simulink model "drone_6dof"  (R2021a)
settings: Solver=VariableStepAuto  StartTime=0.0  StopTime=40  RelTol=1e-3
values from neighbouring files (symbols this model uses):
  controller = designController6DoF(requirements, dynamics)    [mainNelderMead_NOTUSED.m]    (also in mainPSO.m = controllerPre)
  dynamics = getDroneDynamics6DoF()    [mainNelderMead_NOTUSED.m]    (also in mainPSO.m; showResults.m)
undefined symbols (not defined in the file or in its folder): phi0, psi0, theta0, x0, y0, z0
libraries: shared6dof x1
settings Model: SimulationMode=accelerator  Creator=rudog  LastModifiedBy=luizgiacomossi
settings SolverCC: AlgebraicLoopSolver=TrustRegion
settings DebuggingCC: SFMachineParentedDataDiag=warning

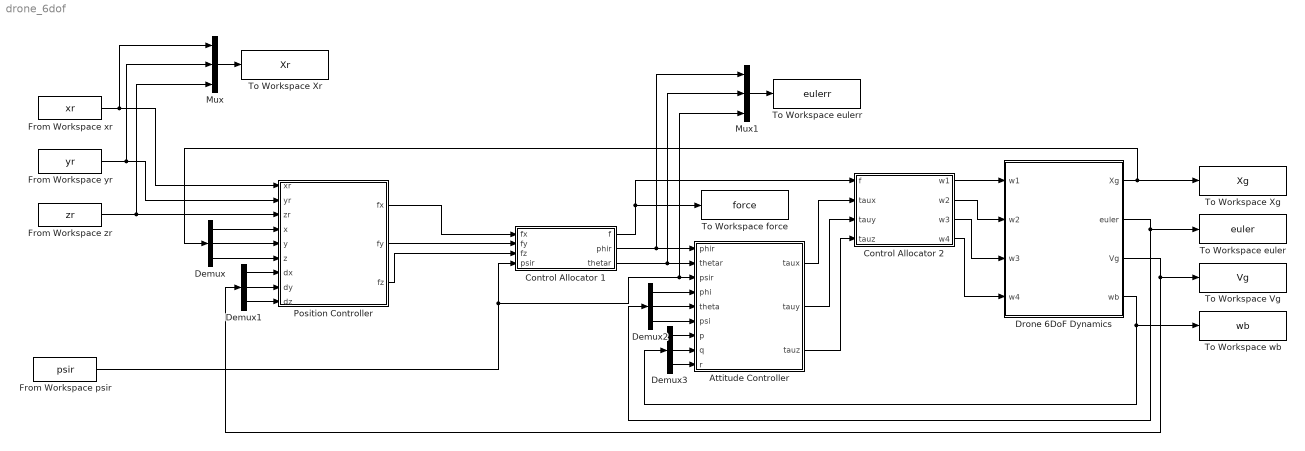
== system drone_6dof ==
  Attitude Controller : Subsystem
  Control Allocator 1 : Subsystem
  Control Allocator 2 : Subsystem
  Demux{,1..3} (4 alike) : Demux  Outputs=3
  Drone 6DoF Dynamics : Subsystem
  From Workspace psir : FromWorkspace  VariableName=psir
  From Workspace xr : FromWorkspace  VariableName=xr
  From Workspace yr : FromWorkspace  VariableName=yr
  From Workspace zr : FromWorkspace  VariableName=zr
  Mux : Mux  Inputs=3
  Mux1 : Mux  Inputs=3
  Position Controller : Subsystem
  To Workspace Vg : ToWorkspace  VariableName=Vg  SaveFormat=Structure With Time  SampleTime=-1
  To Workspace Xg : ToWorkspace  VariableName=Xg  SaveFormat=Structure With Time  SampleTime=-1
  To Workspace Xr : ToWorkspace  VariableName=Xr  SaveFormat=Structure With Time  SampleTime=-1
  To Workspace euler : ToWorkspace  VariableName=euler  SaveFormat=Structure With Time  SampleTime=-1
  To Workspace eulerr : ToWorkspace  VariableName=eulerr  SaveFormat=Structure With Time  SampleTime=-1
  To Workspace force : ToWorkspace  VariableName=force  SaveFormat=Structure With Time  SampleTime=-1
  To Workspace wb : ToWorkspace  VariableName=wb  SaveFormat=Structure With Time  SampleTime=-1
  wires:
  Demux/1 -> Position Controller/4(x)
  Demux/2 -> Position Controller/5(y)
  Demux/3 -> Position Controller/6(z)
  Demux1/1 -> Position Controller/7(dx)
  Demux1/2 -> Position Controller/8(dy)
  Demux1/3 -> Position Controller/9(dz)
  Demux2/1 -> Attitude Controller/4(phi)
  Demux2/2 -> Attitude Controller/5(theta)
  Demux2/3 -> Attitude Controller/6(psi)
  Demux3/1 -> Attitude Controller/7(p)
  Demux3/2 -> Attitude Controller/8(q)
  Demux3/3 -> Attitude Controller/9(r)
  From Workspace zr/1 -> Mux/3, Position Controller/3(zr)
  From Workspace yr/1 -> Mux/2, Position Controller/2(yr)
  From Workspace xr/1 -> Mux/1, Position Controller/1(xr)
  Control Allocator 2/1(w1) -> Drone 6DoF Dynamics/1(w1)
  Control Allocator 2/2(w2) -> Drone 6DoF Dynamics/2(w2)
  Control Allocator 2/3(w3) -> Drone 6DoF Dynamics/3(w3)
  Control Allocator 2/4(w4) -> Drone 6DoF Dynamics/4(w4)
  Control Allocator 1/1(f) -> To Workspace force/1, Control Allocator 2/1(f)
  Attitude Controller/1(taux) -> Control Allocator 2/2(taux)
  Attitude Controller/2(tauy) -> Control Allocator 2/3(tauy)
  Attitude Controller/3(tauz) -> Control Allocator 2/4(tauz)
  Drone 6DoF Dynamics/3(Vg) -> Demux1/1, To Workspace Vg/1
  Drone 6DoF Dynamics/4(wb) -> Demux3/1, To Workspace wb/1
  Mux/1 -> To Workspace Xr/1
  Control Allocator 1/2(phir) -> Mux1/1, Attitude Controller/1(phir)
  Control Allocator 1/3(thetar) -> Mux1/2, Attitude Controller/2(thetar)
  From Workspace psir/1 -> Control Allocator 1/4(psir), Mux1/3, Attitude Controller/3(psir)
  Mux1/1 -> To Workspace eulerr/1
  Position Controller/2(fy) -> Control Allocator 1/2(fy)
  Position Controller/1(fx) -> Control Allocator 1/1(fx)
  Position Controller/3(fz) -> Control Allocator 1/3(fz)
  Drone 6DoF Dynamics/2(euler) -> Demux2/1, To Workspace euler/1
  Drone 6DoF Dynamics/1(Xg) -> To Workspace Xg/1, Demux/1

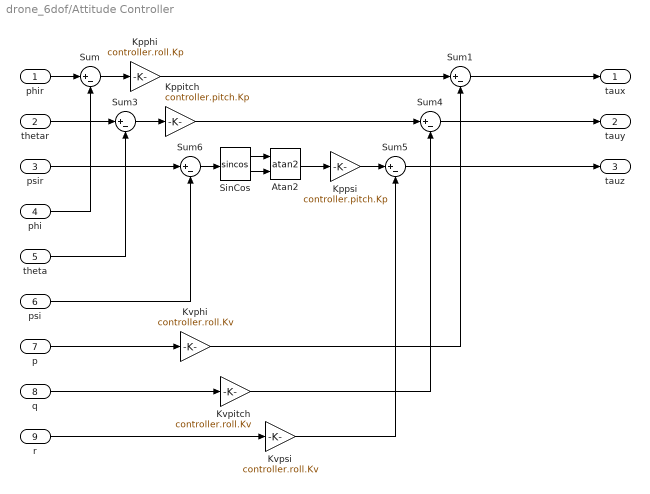
== system drone_6dof/Attitude Controller ==
  phir : Inport
  thetar : Inport  Port=2
  psir : Inport  Port=3
  phi : Inport  Port=4
  theta : Inport  Port=5
  psi : Inport  Port=6
  p : Inport  Port=7
  q : Inport  Port=8
  r : Inport  Port=9
  Atan2 : Trigonometry  Operator=atan2
  Kpphi : Gain  Gain=controller.roll.Kp
  Kppitch : Gain  Gain=controller.pitch.Kp
  Kppsi : Gain  Gain=controller.pitch.Kp
  Kvphi : Gain  Gain=controller.roll.Kv
  Kvpitch : Gain  Gain=controller.roll.Kv
  Kvpsi : Gain  Gain=controller.roll.Kv
  SinCos : Trigonometry  Operator=sincos
  Sum{,1,3..6} (6 alike) : Sum  Inputs=|+-
  taux : Outport
  tauy : Outport  Port=2
  tauz : Outport  Port=3
  wires:
  Kvphi/1 -> Sum1/2
  p/1 -> Kvphi/1
  Kppsi/1 -> Sum5/1
  Sum3/1 -> Kppitch/1
  theta/1 -> Sum3/2
  phir/1 -> Sum/1
  SinCos/1 -> Atan2/1
  Sum1/1 -> taux/1
  Kppitch/1 -> Sum4/1
  Kvpitch/1 -> Sum4/2
  Sum4/1 -> tauy/1
  Kpphi/1 -> Sum1/1
  q/1 -> Kvpitch/1
  r/1 -> Kvpsi/1
  psi/1 -> Sum6/2
  psir/1 -> Sum6/1
  Sum6/1 -> SinCos/1
  SinCos/2 -> Atan2/2
  Sum5/1 -> tauz/1
  Kvpsi/1 -> Sum5/2
  thetar/1 -> Sum3/1
  Atan2/1 -> Kppsi/1
  phi/1 -> Sum/2
  Sum/1 -> Kpphi/1

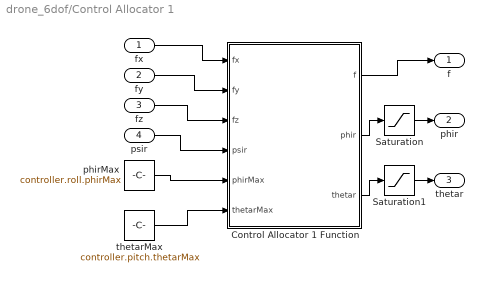
== system drone_6dof/Control Allocator 1 ==
  fx : Inport
  fy : Inport  Port=2
  fz : Inport  Port=3
  psir : Inport  Port=4
  Control Allocator 1 Function : MATLAB Function  TreatAsAtomicUnit=on
  Saturation : Saturate  UpperLimit=30 * pi/180  LowerLimit=- 30 * pi/180
  Saturation1 : Saturate  UpperLimit=30 * pi/180  LowerLimit=- 30 * pi/180
  phirMax : Constant  Value=controller.roll.phirMax
  thetarMax : Constant  Value=controller.pitch.thetarMax
  f : Outport
  phir : Outport  Port=2
  thetar : Outport  Port=3
  wires:
  fx/1 -> Control Allocator 1 Function/1(fx)
  fy/1 -> Control Allocator 1 Function/2(fy)
  fz/1 -> Control Allocator 1 Function/3(fz)
  psir/1 -> Control Allocator 1 Function/4(psir)
  Control Allocator 1 Function/1(f) -> f/1
  Control Allocator 1 Function/2(phir) -> Saturation/1
  Control Allocator 1 Function/3(thetar) -> Saturation1/1
  phirMax/1 -> Control Allocator 1 Function/5(phirMax)
  thetarMax/1 -> Control Allocator 1 Function/6(thetarMax)
  Saturation/1 -> phir/1
  Saturation1/1 -> thetar/1

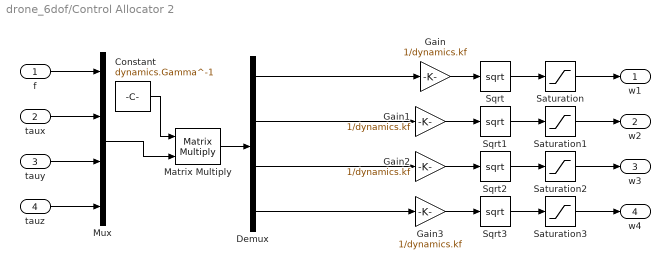
== system drone_6dof/Control Allocator 2 ==
  f : Inport
  taux : Inport  Port=2
  tauy : Inport  Port=3
  tauz : Inport  Port=4
  Constant : Constant  Value=dynamics.Gamma^-1
  Demux : Demux
  Gain{,1..3} (4 alike) : Gain  Gain=1/dynamics.kf
  Matrix Multiply : Product  Multiplication=Matrix(*)
  Mux : Mux
  Saturation{,1..3} (4 alike) : Saturate  UpperLimit=dynamics.wMax  LowerLimit=dynamics.wMin
  Sqrt{,1..3} (4 alike) : Sqrt  SaturateOnIntegerOverflow=on
  w1 : Outport
  w2 : Outport  Port=2
  w3 : Outport  Port=3
  w4 : Outport  Port=4
  wires:
  Gain/1 -> Sqrt/1
  Gain1/1 -> Sqrt1/1
  Gain2/1 -> Sqrt2/1
  Gain3/1 -> Sqrt3/1
  Sqrt3/1 -> Saturation3/1
  Sqrt2/1 -> Saturation2/1
  Sqrt1/1 -> Saturation1/1
  Sqrt/1 -> Saturation/1
  Saturation/1 -> w1/1
  Saturation1/1 -> w2/1
  Saturation2/1 -> w3/1
  Saturation3/1 -> w4/1
  Demux/2 -> Gain1/1
  Demux/4 -> Gain3/1
  Demux/3 -> Gain2/1
  f/1 -> Mux/1
  taux/1 -> Mux/2
  tauy/1 -> Mux/3
  tauz/1 -> Mux/4
  Constant/1 -> Matrix Multiply/1
  Mux/1 -> Matrix Multiply/2
  Matrix Multiply/1 -> Demux/1
  Demux/1 -> Gain/1

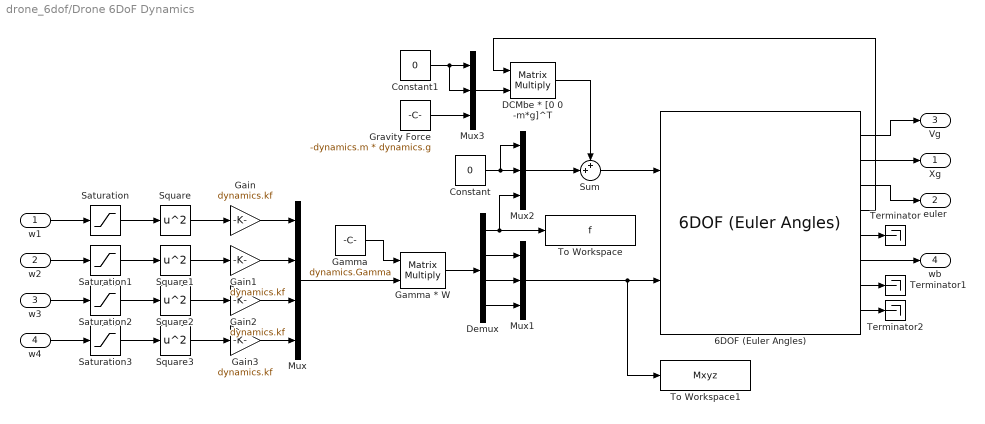
== system drone_6dof/Drone 6DoF Dynamics ==
  w1 : Inport
  w2 : Inport  Port=2
  w3 : Inport  Port=3
  w4 : Inport  Port=4
  6DOF (Euler Angles) : shared6dof/6DOF (Euler Angles)  units=Metric (MKS)  mtype=Fixed  rep=Euler Angles  xme_0=[x0, y0, z0]  Vm_0=[0 0 0]  eul_0=[phi0, theta0, psi0]  pm_0=[0 0 0]  mass_0=dynamics.m  mass_e=0.5  mass_f=2.0  inertia=dynamics.J  inertia_e=eye(3)  inertia_f=2*eye(3)  k_quat=1.0  vre_flag=on  abi_flag=off  aMode=0  xme_statename=''  Vm_statename=''  eul_statename=''  quat_statename=''  pm_statename=''  mass_statename=''
      settings: SourceProductBaseCode=AE,PW,DR,MT,UV,VE
  Constant : Constant  Value=0
  Constant1 : Constant  Value=0
  DCMbe * [0 0 -m*g]^T : Product  Multiplication=Matrix(*)
  Demux : Demux
  Gain{,1..3} (4 alike) : Gain  Gain=dynamics.kf
  Gamma : Constant  Value=dynamics.Gamma
  Gamma * W : Product  Multiplication=Matrix(*)
  Gravity Force : Constant  Value=-dynamics.m * dynamics.g
  Mux : Mux
  Mux1 : Mux  Inputs=3
  Mux2 : Mux  Inputs=3
  Mux3 : Mux  Inputs=3
  Saturation{,1..3} (4 alike) : Saturate  UpperLimit=dynamics.wMax  LowerLimit=dynamics.wMin
  Square{,1..3} (4 alike) : Math  Operator=square  SaturateOnIntegerOverflow=on
  Sum : Sum  Inputs=++|
  Terminator : Terminator
  Terminator1 : Terminator
  Terminator2 : Terminator
  To Workspace : ToWorkspace  VariableName=f  SaveFormat=Structure With Time  SampleTime=-1
  To Workspace1 : ToWorkspace  VariableName=Mxyz  SaveFormat=Structure With Time  SampleTime=-1
  Xg : Outport
  euler : Outport  Port=2
  Vg : Outport  Port=3
  wb : Outport  Port=4
  wires:
  6DOF (Euler Angles)/2 -> Xg/1
  6DOF (Euler Angles)/1 -> Vg/1
  6DOF (Euler Angles)/3 -> euler/1
  w1/1 -> Saturation/1
  w2/1 -> Saturation1/1
  w3/1 -> Saturation2/1
  w4/1 -> Saturation3/1
  Gamma * W/1 -> Demux/1
  Demux/2 -> Mux1/1
  Demux/3 -> Mux1/2
  Demux/4 -> Mux1/3
  Mux1/1 -> To Workspace1/1, 6DOF (Euler Angles)/2
  Mux/1 -> Gamma * W/2
  Gamma/1 -> Gamma * W/1
  Constant/1 -> Mux2/1, Mux2/2
  Demux/1 -> Mux2/3, To Workspace/1
  Mux2/1 -> Sum/2
  Sum/1 -> 6DOF (Euler Angles)/1
  6DOF (Euler Angles)/6 -> wb/1
  6DOF (Euler Angles)/5 -> Terminator/1
  6DOF (Euler Angles)/7 -> Terminator1/1
  6DOF (Euler Angles)/8 -> Terminator2/1
  Gravity Force/1 -> Mux3/3
  Mux3/1 -> DCMbe * [0 0 -m*g]^T/2
  6DOF (Euler Angles)/4 -> DCMbe * [0 0 -m*g]^T/1
  Constant1/1 -> Mux3/2, Mux3/1
  DCMbe * [0 0 -m*g]^T/1 -> Sum/1
  Saturation/1 -> Square/1
  Square/1 -> Gain/1
  Gain/1 -> Mux/1
  Gain1/1 -> Mux/2
  Saturation1/1 -> Square1/1
  Saturation2/1 -> Square2/1
  Saturation3/1 -> Square3/1
  Square1/1 -> Gain1/1
  Square2/1 -> Gain2/1
  Square3/1 -> Gain3/1
  Gain2/1 -> Mux/3
  Gain3/1 -> Mux/4

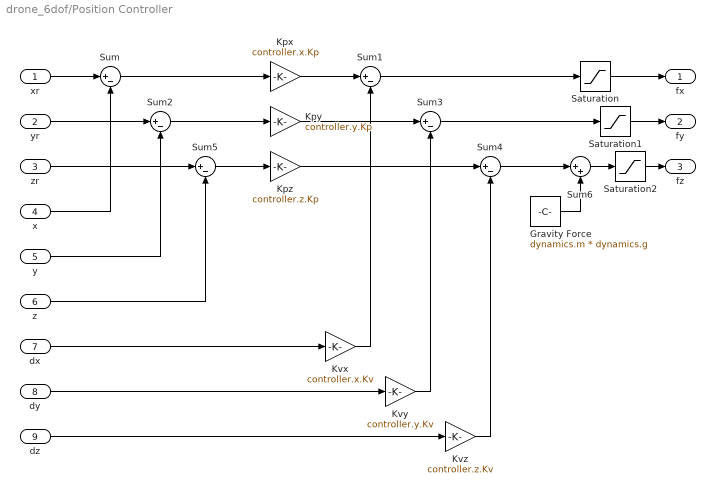
== system drone_6dof/Position Controller ==
  xr : Inport
  yr : Inport  Port=2
  zr : Inport  Port=3
  x : Inport  Port=4
  y : Inport  Port=5
  z : Inport  Port=6
  dx : Inport  Port=7
  dy : Inport  Port=8
  dz : Inport  Port=9
  Gravity Force : Constant  Value=dynamics.m * dynamics.g
  Kpx : Gain  Gain=controller.x.Kp
  Kpy : Gain  Gain=controller.y.Kp
  Kpz : Gain  Gain=controller.z.Kp
  Kvx : Gain  Gain=controller.x.Kv
  Kvy : Gain  Gain=controller.y.Kv
  Kvz : Gain  Gain=controller.z.Kv
  Saturation : Saturate  UpperLimit=controller.x.fMax  LowerLimit=controller.x.fMin
  Saturation1 : Saturate  UpperLimit=controller.y.fMax  LowerLimit=controller.y.fMin
  Saturation2 : Saturate  UpperLimit=controller.z.fMax  LowerLimit=controller.z.fMin
  Sum{,1..5} (6 alike) : Sum  Inputs=|+-
  Sum6 : Sum  Inputs=|++
  fx : Outport
  fy : Outport  Port=2
  fz : Outport  Port=3
  wires:
  xr/1 -> Sum/1
  Kvx/1 -> Sum1/2
  Sum1/1 -> Saturation/1
  Kpz/1 -> Sum4/1
  z/1 -> Sum5/2
  Kpy/1 -> Sum3/1
  Sum3/1 -> Saturation1/1
  y/1 -> Sum2/2
  Sum6/1 -> Saturation2/1
  Kvz/1 -> Sum4/2
  Gravity Force/1 -> Sum6/2
  yr/1 -> Sum2/1
  Kpx/1 -> Sum1/1
  x/1 -> Sum/2
  dx/1 -> Kvx/1
  dz/1 -> Kvz/1
  Kvy/1 -> Sum3/2
  Sum2/1 -> Kpy/1
  zr/1 -> Sum5/1
  Sum4/1 -> Sum6/1
  dy/1 -> Kvy/1
  Sum5/1 -> Kpz/1
  Sum/1 -> Kpx/1
  Saturation/1 -> fx/1
  Saturation1/1 -> fy/1
  Saturation2/1 -> fz/1

== matlab function drone_6dof/Control Allocator 1/Control Allocator 1 Function ==
  data: f output; phir output; thetar output; fx input; fy input; fz input; psir input; phirMax input; thetarMax input
function [f, phir, thetar] = controlAllocator1(fx, fy, fz, psir, phirMax,thetarMax)
% [f, phir, thetar] = controlAllocator1(fx, fy, fz, psir, phirMax,
% thetarMax) implements a control allocator that computes roll and pitch
% references phir and thetar along with the vertical force generated by the
% propellers to attain a desired force vector [fx, fy, fz]^T. The inputs
% are:
% fx: x component of the desired force.
% fy: y component of the desired force.
% fz: z component of the desired force.
% psir: reference yaw angle.
% phirMax: phir is saturated to stay within [-phirMax, phirMax].
% thetarMax: thetar is saturated to stay within [-thetarMax, thetarMax].

% Implement



f = norm([fx; fy; fz]);

nx = fx/f;
ny = fy/f;
nz = fz/f;


phir = asin(nx*sin(psir)-ny*cos(psir));

thetar = atan2(nx*cos(psir)+ny*sin(psir),nz);
